simulink model "modelo_rhex_tripode_alterno"  (R2020a)
settings: Solver=VariableStepAuto  StartTime=0.0  StopTime=10.0  RelTol=1e-3
values from neighbouring files (symbols this model uses):
  dist1 = 275    [Parametros_RHex.m]
  espesor = 10    [Parametros_RHex.m]
  masa_C_Leg = 0.057    [Parametros_RHex.m]
  radio = 100    [Parametros_RHex.m]
undefined symbols (not defined in the file or in its folder): X, Y, Z
libraries: sm_lib x34, Contact_Forces_Lib x22, nesl_utility x19, simulink x1
(part 2 of 2)

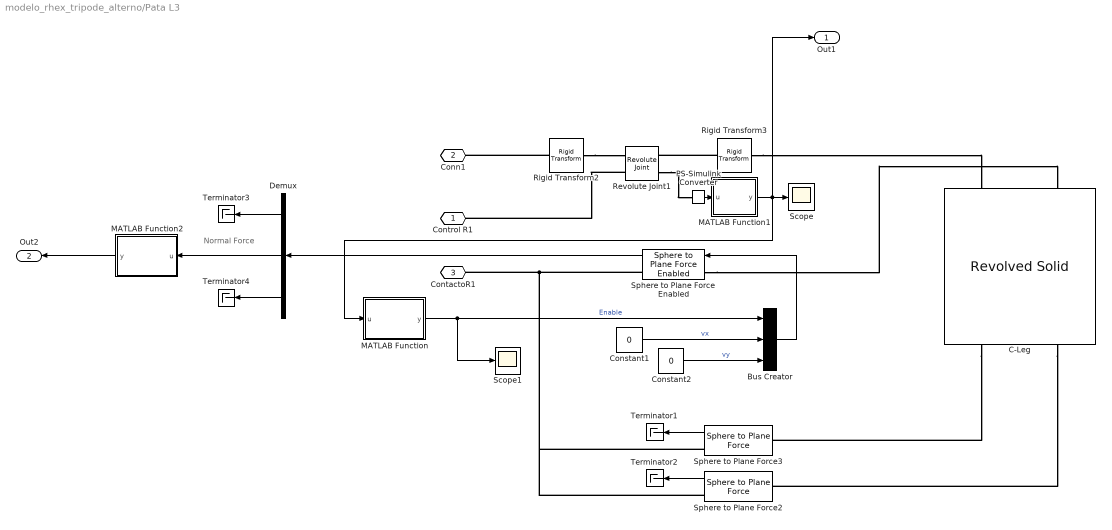
== system modelo_rhex_tripode_alterno/Pata L3 ==
  note: Normal Force
  Bus Creator : BusCreator  Inputs=3
  C-Leg : sm_lib/Body Elements/Revolved Solid  GraphicAmbientColor=[0.15 0.15 0.15 1.0]  BasedOnType=Mass  CenterOfMass=[-42.439/1000 25/1000 -108.743/1000]  CenterOfMassUnits=mm  GraphicDiffuseColor=[1.0 0.2 0.0]  ExportConvexHullGeometry=off  Density=1000  DensityUnits=kg/m^3  DoExposeReferenceFrame=on  GraphicEmissiveColor=[0.0 0.0 0.0 1.0]  ExportEntireGeometry=off  SerializedFrames=<Frames><Frame><Id>Frame1</Id><Value><Name>F1</Name><Origin><Source>GeometricFeature</Source><FeatureName>front point 2</FeatureName></Origin><PrimaryAxis><DefinedDirection>+Z</DefinedDirection><Source>ReferenceFrame</Source><SourceDirection>+Z</SourceDirection><FeatureName></FeatureName></PrimaryAxis><SecondaryAxis><DefinedDirection>+X</DefinedDirection><Source>ReferenceFrame</Source><SourceDirection>+X</SourceDirection><FeatureName></FeatureName></SecondaryAxis></Value></Frame><Frame><Id>Frame2</Id><Value><Name>F2</Name><Origin><Source>GeometricFeature</Source><FeatureName>front point 3</FeatureName></Origin><PrimaryAxis><DefinedDirection>+Z</DefinedDirection><Source>ReferenceFrame</Source><SourceDirection>+Z</SourceDirection><FeatureName></FeatureName></PrimaryAxis><SecondaryAxis><DefinedDirection>+X</DefinedDirection><Source>ReferenceFrame</Source><SourceDirection>+X</SourceDirection><FeatureName></FeatureName></SecondaryAxis></Value></Frame><Frame><Id>Frame3</Id><Value><Name>F3</Name><Origin><Source>GeometricFeature</Source><FeatureName>side surface 2</FeatureName></Origin><PrimaryAxis><DefinedDirection>+Z</DefinedDirection><Source>ReferenceFrame</Source><SourceDirection>+Z</SourceDirection><FeatureName></FeatureName></PrimaryAxis><SecondaryAxis><DefinedDirection>+X</DefinedDirection><Source>ReferenceFrame</Source><SourceDirection>+X</SourceDirection><FeatureName></FeatureName></SecondaryAxis></Value></Frame></Frames>  MarkerShape=Sphere  MarkerSize=10  GraphicType=FromGeometry  InertiaType=Custom  Mass=masa_C_Leg  MassUnits=kg  MomentsOfInertia=[0.001038176 0.000273753 0.001217746]  MomentsOfInertiaUnits=kg*mm^2  GraphicOpacity=1.0  ProductsOfInertia=[-0.000218169 0.000059956 0.000153627]  ProductsOfInertiaUnits=kg*mm^2  RevolutionCrossSection=perfil_C_Leg  RevolutionCrossSectionUnits=mm  RevolutionAngle=240  RevolutionAngleUnits=deg  RevolutionExtent=Custom  GraphicShininess=75  GraphicSpecularColor=[0.5 0.5 0.5 1.0]  GraphicVisPropType=SimpleVisualProperties
  Constant1 : Constant  Value=0
  Constant2 : Constant  Value=0
  Demux : Demux  Outputs=3
  MATLAB Function : MATLAB Function  TreatAsAtomicUnit=on
  MATLAB Function1 : MATLAB Function  TreatAsAtomicUnit=on
  MATLAB Function2 : MATLAB Function  TreatAsAtomicUnit=on
  PS-Simulink Converter : nesl_utility/PS-Simulink Converter  PhysicalDomain=network_engine_domain  SubClassName=ps_output  LeftPortType=input  RightPortType=output  PseudoPeriodic=off  Frequencies=[]  Unit=rad  AffineConversion=off
  Revolute Joint1 : sm_lib/Joints/Revolute Joint  JointMode=Normal  SenseConstraintForce=off  SenseConstraintForceX=off  SenseConstraintForceY=off  SenseConstraintForceZ=off  SenseConstraintTorque=off  SenseConstraintTorqueX=off  SenseConstraintTorqueY=off  SenseConstraintTorqueZ=off  SenseTotalForce=off  SenseTotalForceX=off  SenseTotalForceY=off  SenseTotalForceZ=off  SenseTotalTorque=off  SenseTotalTorqueX=off  SenseTotalTorqueY=off  SenseTotalTorqueZ=off  CompositeWrenchDir=FollowerOnBase  CompositeWrenchFrame=BaseFrame  EquilibriumPosition=0  EquilibriumPositionUnits=deg  SpringStiffness=0  SpringStiffnessUnits=N*m/deg  DampingCoefficient=0  DampingCoefficientUnits=N*m/(deg/s)  TorqueActuationMode=ComputedTorque  MotionActuationMode=InputMotion  SensePosition=on  SenseVelocity=off  SenseAcceleration=off  SenseTorqueForce=off  SenseLowerLimitTorqueForce=off  SenseUpperLimitTorqueForce=off  LowerLimitSpecify=off  LowerLimitBound=-90  LowerLimitBoundUnits=deg  LowerLimitStiffness=1e4  LowerLimitStiffnessUnits=N*m/deg  LowerLimitDamping=10  LowerLimitDampingUnits=N*m/(deg/s)  LowerLimitTransitionRegionWidth=0.1  LowerLimitTransitionRegionWidthUnits=deg  UpperLimitSpecify=off  UpperLimitBound=90  UpperLimitBoundUnits=deg  UpperLimitStiffness=1e4  UpperLimitStiffnessUnits=N*m/deg  UpperLimitDamping=10  UpperLimitDampingUnits=N*m/(deg/s)  UpperLimitTransitionRegionWidth=0.1  UpperLimitTransitionRegionWidthUnits=deg  PositionTargetSpecify=on  PositionTargetPriority=High  PositionTargetValue=180  PositionTargetValueUnits=deg  VelocityTargetSpecify=off  VelocityTargetPriority=High  VelocityTargetValue=0  VelocityTargetValueUnits=deg/s
  Rigid Transform2 : sm_lib/Frames and Transforms/Rigid Transform  TranslationMethod=Cartesian  TranslationStandardOffset=dist4  TranslationLengthUnit=cm  TranslationStandardAxis=+Y  TranslationCartesianOffset=[-23.635 27.496 0]  TranslationROffset=0  TranslationROffsetUnits=m  TranslationZOffset=0  TranslationZOffsetUnits=m  TranslationThetaOffset=0  TranslationThetaOffsetUnits=deg  RotationMethod=StandardAxis  RotationAngleUnits=deg  RotationStandardAxis=+X  RotationAngle=90  RotationArbitraryAxis=[0 0 1]  FollAlignAxisA=-Z  BaseAlignAxisA=+X  FollAlignAxisB=+X  BaseAlignAxisB=+Z  RotationSequenceAxes=FollowerAxes  RotationSequence=XYX  RotationSequenceAngles=[0 0 0]  RotationSequenceAnglesUnits=deg  RotationMatrix=[1 0 0; 0 1 0; 0 0 1]
  Rigid Transform3 : sm_lib/Frames and Transforms/Rigid Transform  TranslationMethod=Cylindrical  TranslationStandardOffset=0  TranslationLengthUnit=mm  TranslationStandardAxis=+Z  TranslationCartesianOffset=[0 -(dist1/2)-radio+(espesor/2) 0]  TranslationROffset=radio-espesor/2  TranslationROffsetUnits=mm  TranslationZOffset=0  TranslationZOffsetUnits=m  TranslationThetaOffset=-120  TranslationThetaOffsetUnits=deg  RotationMethod=StandardAxis  RotationAngleUnits=deg  RotationStandardAxis=+Z  RotationAngle=0  RotationArbitraryAxis=[0 0 1]  FollAlignAxisA=-Z  BaseAlignAxisA=+X  FollAlignAxisB=+X  BaseAlignAxisB=+Z  RotationSequenceAxes=FollowerAxes  RotationSequence=XYX  RotationSequenceAngles=[0 0 0]  RotationSequenceAnglesUnits=deg  RotationMatrix=[1 0 0; 0 1 0; 0 0 1]
  Scope : Scope
  Scope1 : Scope
  Sphere to Plane Force Enabled : Contact_Forces_Lib/3D/Sphere to Plane Force Enabled  sphere_rad=radio/1000  plane_lenx=10  plane_leny=10  plane_depth=0.05/2  force_law=Linear  k_contact=cont1  b_contact=cont2  pen_full_damp_F=0  pen_exponent=1  custom_param_1=1  custom_param_2=1  friction_law=Stick-Slip Continuous  mu_kinetic=fric1  mu_static=fric2  v_thr=0.1  vis_on=off  vis_opc_en=0  vis_len_plaBz=0.005  vis_clr=[0.9 0.2 0.2]  vis_opc=0.7
      settings: SourceProductName=Simscape Multibody Contact Forces Library
  Sphere to Plane Force2 : Contact_Forces_Lib/3D/Sphere to Plane Force  sphere_rad=1e-6  plane_lenx=10  plane_leny=10  plane_depth=0.025  force_law=Linear  k_contact=cont1  b_contact=cont2  pen_full_damp_F=1e-4  pen_exponent=1  custom_param_1=1  custom_param_2=1  friction_law=Stick-Slip Continuous  mu_kinetic=fric1  mu_static=fric2  v_thr=0.1  vis_on=off  vis_opc_en=0  vis_len_plaBz=0.005  vis_clr=[0.9 0.2 0.2]  vis_opc=0.7
  Sphere to Plane Force3 : Contact_Forces_Lib/3D/Sphere to Plane Force  sphere_rad=1e-6  plane_lenx=10  plane_leny=10  plane_depth=0.025  force_law=Linear  k_contact=cont1  b_contact=cont2  pen_full_damp_F=1e-4  pen_exponent=1  custom_param_1=1  custom_param_2=1  friction_law=Stick-Slip Continuous  mu_kinetic=fric1  mu_static=fric2  v_thr=0.1  vis_on=off  vis_opc_en=0  vis_len_plaBz=0.005  vis_clr=[0.9 0.2 0.2]  vis_opc=0.7
  Terminator{1..4} (4 alike) : Terminator
  Control R1 : PMIOPort  Side=Right
  Conn1 : PMIOPort  Port=2  Side=Left
  ContactoR1 : PMIOPort  Port=3  Side=Right
  Out1 : Outport  VectorParamsAs1DForOutWhenUnconnected=off
  Out2 : Outport  Port=2  VectorParamsAs1DForOutWhenUnconnected=off
  wires:
  Constant1/1 -> Bus Creator/2  "vx"
  Constant2/1 -> Bus Creator/3  "vy"
  MATLAB Function/1(y) -> Scope1/1, Bus Creator/1  "Enable"
  PS-Simulink Converter/1 -> MATLAB Function1/1(u)
  MATLAB Function1/1(y) -> Out1/1, MATLAB Function/1(u), Scope/1
  Sphere to Plane Force2/1 -> Terminator2/1
  Sphere to Plane Force3/1 -> Terminator1/1
  Bus Creator/1 -> Sphere to Plane Force Enabled/1
  Demux/1 -> Terminator3/1
  Demux/2 -> MATLAB Function2/1(u)
  Demux/3 -> Terminator4/1
  Sphere to Plane Force Enabled/1 -> Demux/1
  MATLAB Function2/1(y) -> Out2/1
  connections:
  Rigid Transform3/LConn1 -- C-Leg/RConn1
  Rigid Transform3/RConn1 -- Revolute Joint1/RConn1
  Rigid Transform2/LConn1 -- Conn1/RConn1
  Revolute Joint1/LConn2 -- Control R1/RConn1
  Revolute Joint1/RConn2 -- PS-Simulink Converter/LConn1
  C-Leg/LConn1 -- Sphere to Plane Force3/LConn1
  Rigid Transform2/RConn1 -- Revolute Joint1/LConn1
  Sphere to Plane Force2/RConn1 -- Sphere to Plane Force3/RConn1 -- Sphere to Plane Force Enabled/RConn1 -- ContactoR1/RConn1
  C-Leg/LConn2 -- Sphere to Plane Force2/LConn1
  Sphere to Plane Force Enabled/LConn1 -- C-Leg/RConn2

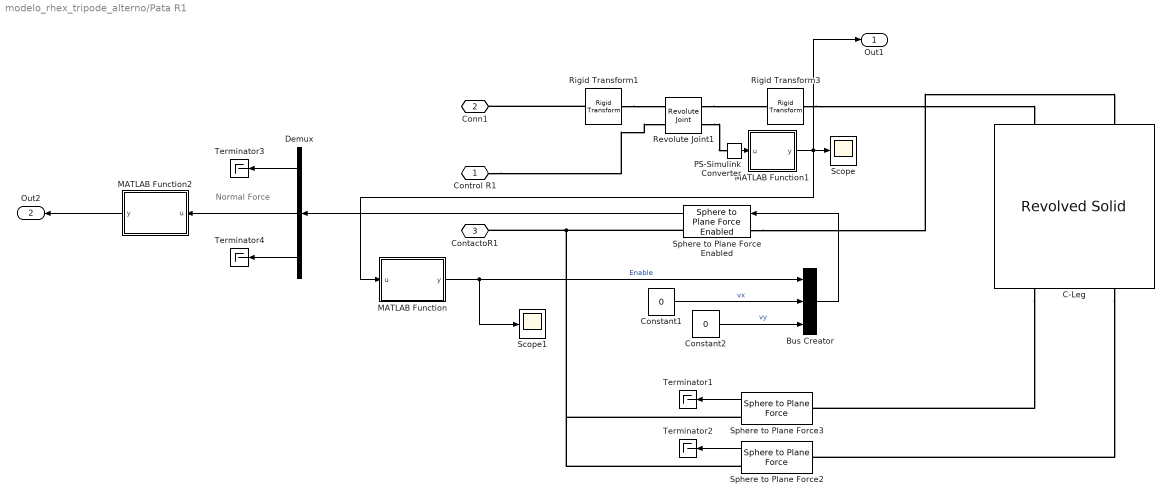
== system modelo_rhex_tripode_alterno/Pata R1 ==
  note: Normal Force
  Bus Creator : BusCreator  Inputs=3
  C-Leg : sm_lib/Body Elements/Revolved Solid  GraphicAmbientColor=[0.15 0.15 0.15 1.0]  BasedOnType=Mass  CenterOfMass=[-42.439/1000 25/1000 -108.743/1000]  CenterOfMassUnits=mm  GraphicDiffuseColor=[1.0 0.2 0.0]  ExportConvexHullGeometry=off  Density=1000  DensityUnits=kg/m^3  DoExposeReferenceFrame=on  GraphicEmissiveColor=[0.0 0.0 0.0 1.0]  ExportEntireGeometry=off  SerializedFrames=<Frames><Frame><Id>Frame1</Id><Value><Name>F1</Name><Origin><Source>GeometricFeature</Source><FeatureName>front point 2</FeatureName></Origin><PrimaryAxis><DefinedDirection>+Z</DefinedDirection><Source>ReferenceFrame</Source><SourceDirection>+Z</SourceDirection><FeatureName></FeatureName></PrimaryAxis><SecondaryAxis><DefinedDirection>+X</DefinedDirection><Source>ReferenceFrame</Source><SourceDirection>+X</SourceDirection><FeatureName></FeatureName></SecondaryAxis></Value></Frame><Frame><Id>Frame2</Id><Value><Name>F2</Name><Origin><Source>GeometricFeature</Source><FeatureName>front point 3</FeatureName></Origin><PrimaryAxis><DefinedDirection>+Z</DefinedDirection><Source>ReferenceFrame</Source><SourceDirection>+Z</SourceDirection><FeatureName></FeatureName></PrimaryAxis><SecondaryAxis><DefinedDirection>+X</DefinedDirection><Source>ReferenceFrame</Source><SourceDirection>+X</SourceDirection><FeatureName></FeatureName></SecondaryAxis></Value></Frame><Frame><Id>Frame3</Id><Value><Name>F3</Name><Origin><Source>GeometricFeature</Source><FeatureName>side surface 2</FeatureName></Origin><PrimaryAxis><DefinedDirection>+Z</DefinedDirection><Source>ReferenceFrame</Source><SourceDirection>+Z</SourceDirection><FeatureName></FeatureName></PrimaryAxis><SecondaryAxis><DefinedDirection>+X</DefinedDirection><Source>ReferenceFrame</Source><SourceDirection>+X</SourceDirection><FeatureName></FeatureName></SecondaryAxis></Value></Frame></Frames>  MarkerShape=Sphere  MarkerSize=10  GraphicType=FromGeometry  InertiaType=Custom  Mass=masa_C_Leg  MassUnits=kg  MomentsOfInertia=[0.001038176 0.000273753 0.001217746]  MomentsOfInertiaUnits=kg*mm^2  GraphicOpacity=1.0  ProductsOfInertia=[-0.000218169 0.000059956 0.000153627]  ProductsOfInertiaUnits=kg*mm^2  RevolutionCrossSection=perfil_C_Leg  RevolutionCrossSectionUnits=mm  RevolutionAngle=240  RevolutionAngleUnits=deg  RevolutionExtent=Custom  GraphicShininess=75  GraphicSpecularColor=[0.5 0.5 0.5 1.0]  GraphicVisPropType=SimpleVisualProperties
  Constant1 : Constant  Value=0
  Constant2 : Constant  Value=0
  Demux : Demux  Outputs=3
  MATLAB Function : MATLAB Function  TreatAsAtomicUnit=on
  MATLAB Function1 : MATLAB Function  TreatAsAtomicUnit=on
  MATLAB Function2 : MATLAB Function  TreatAsAtomicUnit=on
  PS-Simulink Converter : nesl_utility/PS-Simulink Converter  PhysicalDomain=network_engine_domain  SubClassName=ps_output  LeftPortType=input  RightPortType=output  PseudoPeriodic=off  Frequencies=[]  Unit=rad  AffineConversion=off
  Revolute Joint1 : sm_lib/Joints/Revolute Joint  JointMode=Normal  SenseConstraintForce=off  SenseConstraintForceX=off  SenseConstraintForceY=off  SenseConstraintForceZ=off  SenseConstraintTorque=off  SenseConstraintTorqueX=off  SenseConstraintTorqueY=off  SenseConstraintTorqueZ=off  SenseTotalForce=off  SenseTotalForceX=off  SenseTotalForceY=off  SenseTotalForceZ=off  SenseTotalTorque=off  SenseTotalTorqueX=off  SenseTotalTorqueY=off  SenseTotalTorqueZ=off  CompositeWrenchDir=FollowerOnBase  CompositeWrenchFrame=BaseFrame  EquilibriumPosition=0  EquilibriumPositionUnits=deg  SpringStiffness=0  SpringStiffnessUnits=N*m/deg  DampingCoefficient=0  DampingCoefficientUnits=N*m/(deg/s)  TorqueActuationMode=ComputedTorque  MotionActuationMode=InputMotion  SensePosition=on  SenseVelocity=off  SenseAcceleration=off  SenseTorqueForce=off  SenseLowerLimitTorqueForce=off  SenseUpperLimitTorqueForce=off  LowerLimitSpecify=off  LowerLimitBound=-90  LowerLimitBoundUnits=deg  LowerLimitStiffness=1e4  LowerLimitStiffnessUnits=N*m/deg  LowerLimitDamping=10  LowerLimitDampingUnits=N*m/(deg/s)  LowerLimitTransitionRegionWidth=0.1  LowerLimitTransitionRegionWidthUnits=deg  UpperLimitSpecify=off  UpperLimitBound=90  UpperLimitBoundUnits=deg  UpperLimitStiffness=1e4  UpperLimitStiffnessUnits=N*m/deg  UpperLimitDamping=10  UpperLimitDampingUnits=N*m/(deg/s)  UpperLimitTransitionRegionWidth=0.1  UpperLimitTransitionRegionWidthUnits=deg  PositionTargetSpecify=on  PositionTargetPriority=High  PositionTargetValue=180  PositionTargetValueUnits=deg  VelocityTargetSpecify=off  VelocityTargetPriority=High  VelocityTargetValue=0  VelocityTargetValueUnits=deg/s
  Rigid Transform1 : sm_lib/Frames and Transforms/Rigid Transform  TranslationMethod=Cartesian  TranslationStandardOffset=dist4  TranslationLengthUnit=cm  TranslationStandardAxis=+Y  TranslationCartesianOffset=[23.635 -22.425 0]  TranslationROffset=0  TranslationROffsetUnits=m  TranslationZOffset=0  TranslationZOffsetUnits=m  TranslationThetaOffset=0  TranslationThetaOffsetUnits=deg  RotationMethod=StandardAxis  RotationAngleUnits=deg  RotationStandardAxis=+X  RotationAngle=90  RotationArbitraryAxis=[0 0 1]  FollAlignAxisA=-Z  BaseAlignAxisA=+X  FollAlignAxisB=+X  BaseAlignAxisB=+Z  RotationSequenceAxes=FollowerAxes  RotationSequence=XYX  RotationSequenceAngles=[0 0 0]  RotationSequenceAnglesUnits=deg  RotationMatrix=[1 0 0; 0 1 0; 0 0 1]
  Rigid Transform3 : sm_lib/Frames and Transforms/Rigid Transform  TranslationMethod=Cylindrical  TranslationStandardOffset=0  TranslationLengthUnit=mm  TranslationStandardAxis=+Z  TranslationCartesianOffset=[0 -(dist1/2)-radio+(espesor/2) 0]  TranslationROffset=radio-espesor/2  TranslationROffsetUnits=mm  TranslationZOffset=0  TranslationZOffsetUnits=m  TranslationThetaOffset=-120  TranslationThetaOffsetUnits=deg  RotationMethod=StandardAxis  RotationAngleUnits=deg  RotationStandardAxis=+Z  RotationAngle=0  RotationArbitraryAxis=[0 0 1]  FollAlignAxisA=-Z  BaseAlignAxisA=+X  FollAlignAxisB=+X  BaseAlignAxisB=+Z  RotationSequenceAxes=FollowerAxes  RotationSequence=XYX  RotationSequenceAngles=[0 0 0]  RotationSequenceAnglesUnits=deg  RotationMatrix=[1 0 0; 0 1 0; 0 0 1]
  Scope : Scope
  Scope1 : Scope
  Sphere to Plane Force Enabled : Contact_Forces_Lib/3D/Sphere to Plane Force Enabled  sphere_rad=radio/1000  plane_lenx=10  plane_leny=10  plane_depth=0.05/2  force_law=Linear  k_contact=cont1  b_contact=cont2  pen_full_damp_F=0  pen_exponent=1  custom_param_1=1  custom_param_2=1  friction_law=Stick-Slip Continuous  mu_kinetic=fric1  mu_static=fric2  v_thr=0.1  vis_on=off  vis_opc_en=0  vis_len_plaBz=0.005  vis_clr=[0.9 0.2 0.2]  vis_opc=0.7
      settings: SourceProductName=Simscape Multibody Contact Forces Library
  Sphere to Plane Force2 : Contact_Forces_Lib/3D/Sphere to Plane Force  sphere_rad=1e-6  plane_lenx=10  plane_leny=10  plane_depth=0.025  force_law=Linear  k_contact=cont1  b_contact=cont2  pen_full_damp_F=1e-4  pen_exponent=1  custom_param_1=1  custom_param_2=1  friction_law=Stick-Slip Continuous  mu_kinetic=fric1  mu_static=fric2  v_thr=0.1  vis_on=off  vis_opc_en=0  vis_len_plaBz=0.005  vis_clr=[0.9 0.2 0.2]  vis_opc=0.7
  Sphere to Plane Force3 : Contact_Forces_Lib/3D/Sphere to Plane Force  sphere_rad=1e-6  plane_lenx=10  plane_leny=10  plane_depth=0.025  force_law=Linear  k_contact=cont1  b_contact=cont2  pen_full_damp_F=1e-4  pen_exponent=1  custom_param_1=1  custom_param_2=1  friction_law=Stick-Slip Continuous  mu_kinetic=fric1  mu_static=fric2  v_thr=0.1  vis_on=off  vis_opc_en=0  vis_len_plaBz=0.005  vis_clr=[0.9 0.2 0.2]  vis_opc=0.7
  Terminator{1..4} (4 alike) : Terminator
  Control R1 : PMIOPort  Side=Right
  Conn1 : PMIOPort  Port=2  Side=Left
  ContactoR1 : PMIOPort  Port=3  Side=Right
  Out1 : Outport  VectorParamsAs1DForOutWhenUnconnected=off
  Out2 : Outport  Port=2  VectorParamsAs1DForOutWhenUnconnected=off
  wires:
  Constant1/1 -> Bus Creator/2  "vx"
  Constant2/1 -> Bus Creator/3  "vy"
  MATLAB Function/1(y) -> Scope1/1, Bus Creator/1  "Enable"
  PS-Simulink Converter/1 -> MATLAB Function1/1(u)
  MATLAB Function1/1(y) -> Out1/1, MATLAB Function/1(u), Scope/1
  Sphere to Plane Force2/1 -> Terminator2/1
  Sphere to Plane Force3/1 -> Terminator1/1
  Bus Creator/1 -> Sphere to Plane Force Enabled/1
  Demux/1 -> Terminator3/1
  Demux/2 -> MATLAB Function2/1(u)
  Demux/3 -> Terminator4/1
  Sphere to Plane Force Enabled/1 -> Demux/1
  MATLAB Function2/1(y) -> Out2/1
  connections:
  Rigid Transform3/LConn1 -- C-Leg/RConn1
  Rigid Transform1/LConn1 -- Conn1/RConn1
  Control R1/RConn1 -- Revolute Joint1/LConn2
  Sphere to Plane Force2/RConn1 -- Sphere to Plane Force3/RConn1 -- Sphere to Plane Force Enabled/RConn1 -- ContactoR1/RConn1
  C-Leg/LConn1 -- Sphere to Plane Force3/LConn1
  C-Leg/LConn2 -- Sphere to Plane Force2/LConn1
  Revolute Joint1/RConn2 -- PS-Simulink Converter/LConn1
  Revolute Joint1/RConn1 -- Rigid Transform3/RConn1
  Rigid Transform1/RConn1 -- Revolute Joint1/LConn1
  Sphere to Plane Force Enabled/LConn1 -- C-Leg/RConn2

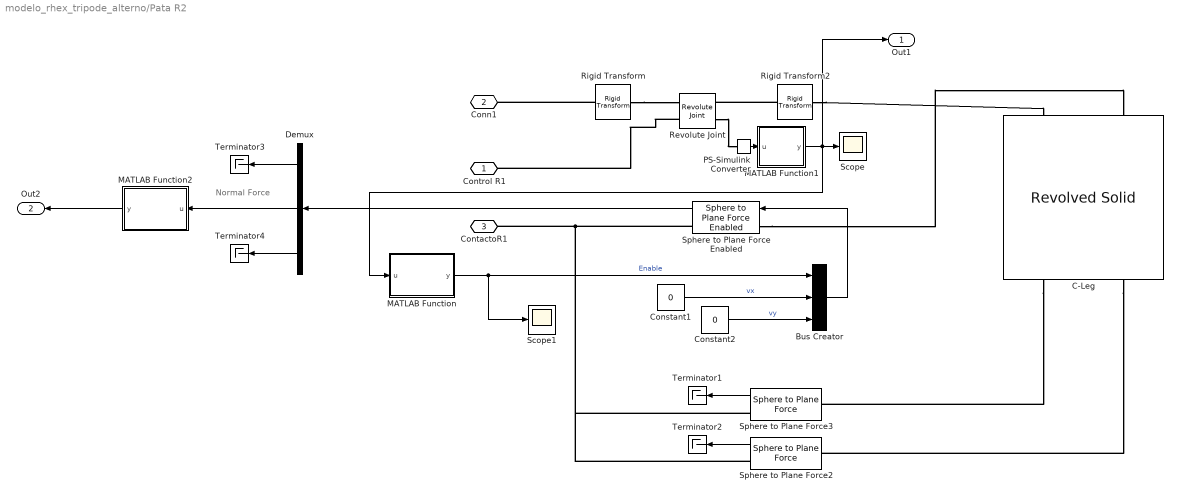
== system modelo_rhex_tripode_alterno/Pata R2 ==
  note: Normal Force
  Bus Creator : BusCreator  Inputs=3
  C-Leg : sm_lib/Body Elements/Revolved Solid  GraphicAmbientColor=[0.15 0.15 0.15 1.0]  BasedOnType=Mass  CenterOfMass=[-42.439/1000 25/1000 -108.743/1000]  CenterOfMassUnits=mm  GraphicDiffuseColor=[1.0 0.2 0.0]  ExportConvexHullGeometry=off  Density=1000  DensityUnits=kg/m^3  DoExposeReferenceFrame=on  GraphicEmissiveColor=[0.0 0.0 0.0 1.0]  ExportEntireGeometry=off  SerializedFrames=<Frames><Frame><Id>Frame1</Id><Value><Name>F1</Name><Origin><Source>GeometricFeature</Source><FeatureName>front point 2</FeatureName></Origin><PrimaryAxis><DefinedDirection>+Z</DefinedDirection><Source>ReferenceFrame</Source><SourceDirection>+Z</SourceDirection><FeatureName></FeatureName></PrimaryAxis><SecondaryAxis><DefinedDirection>+X</DefinedDirection><Source>ReferenceFrame</Source><SourceDirection>+X</SourceDirection><FeatureName></FeatureName></SecondaryAxis></Value></Frame><Frame><Id>Frame2</Id><Value><Name>F2</Name><Origin><Source>GeometricFeature</Source><FeatureName>front point 3</FeatureName></Origin><PrimaryAxis><DefinedDirection>+Z</DefinedDirection><Source>ReferenceFrame</Source><SourceDirection>+Z</SourceDirection><FeatureName></FeatureName></PrimaryAxis><SecondaryAxis><DefinedDirection>+X</DefinedDirection><Source>ReferenceFrame</Source><SourceDirection>+X</SourceDirection><FeatureName></FeatureName></SecondaryAxis></Value></Frame><Frame><Id>Frame3</Id><Value><Name>F3</Name><Origin><Source>GeometricFeature</Source><FeatureName>side surface 2</FeatureName></Origin><PrimaryAxis><DefinedDirection>+Z</DefinedDirection><Source>ReferenceFrame</Source><SourceDirection>+Z</SourceDirection><FeatureName></FeatureName></PrimaryAxis><SecondaryAxis><DefinedDirection>+X</DefinedDirection><Source>ReferenceFrame</Source><SourceDirection>+X</SourceDirection><FeatureName></FeatureName></SecondaryAxis></Value></Frame></Frames>  MarkerShape=Sphere  MarkerSize=10  GraphicType=FromGeometry  InertiaType=Custom  Mass=masa_C_Leg  MassUnits=kg  MomentsOfInertia=[0.001038176 0.000273753 0.001217746]  MomentsOfInertiaUnits=kg*mm^2  GraphicOpacity=1.0  ProductsOfInertia=[-0.000218169 0.000059956 0.000153627]  ProductsOfInertiaUnits=kg*mm^2  RevolutionCrossSection=perfil_C_Leg  RevolutionCrossSectionUnits=mm  RevolutionAngle=240  RevolutionAngleUnits=deg  RevolutionExtent=Custom  GraphicShininess=75  GraphicSpecularColor=[0.5 0.5 0.5 1.0]  GraphicVisPropType=SimpleVisualProperties
  Constant1 : Constant  Value=0
  Constant2 : Constant  Value=0
  Demux : Demux  Outputs=3
  MATLAB Function : MATLAB Function  TreatAsAtomicUnit=on
  MATLAB Function1 : MATLAB Function  TreatAsAtomicUnit=on
  MATLAB Function2 : MATLAB Function  TreatAsAtomicUnit=on
  PS-Simulink Converter : nesl_utility/PS-Simulink Converter  PhysicalDomain=network_engine_domain  SubClassName=ps_output  LeftPortType=input  RightPortType=output  PseudoPeriodic=off  Frequencies=[]  Unit=rad  AffineConversion=off
  Revolute Joint : sm_lib/Joints/Revolute Joint  JointMode=Normal  SenseConstraintForce=off  SenseConstraintForceX=off  SenseConstraintForceY=off  SenseConstraintForceZ=off  SenseConstraintTorque=off  SenseConstraintTorqueX=off  SenseConstraintTorqueY=off  SenseConstraintTorqueZ=off  SenseTotalForce=off  SenseTotalForceX=off  SenseTotalForceY=off  SenseTotalForceZ=off  SenseTotalTorque=off  SenseTotalTorqueX=off  SenseTotalTorqueY=off  SenseTotalTorqueZ=off  CompositeWrenchDir=FollowerOnBase  CompositeWrenchFrame=BaseFrame  EquilibriumPosition=0  EquilibriumPositionUnits=deg  SpringStiffness=0  SpringStiffnessUnits=N*m/deg  DampingCoefficient=0  DampingCoefficientUnits=N*m/(deg/s)  TorqueActuationMode=ComputedTorque  MotionActuationMode=InputMotion  SensePosition=on  SenseVelocity=off  SenseAcceleration=off  SenseTorqueForce=off  SenseLowerLimitTorqueForce=off  SenseUpperLimitTorqueForce=off  LowerLimitSpecify=off  LowerLimitBound=-90  LowerLimitBoundUnits=deg  LowerLimitStiffness=1e4  LowerLimitStiffnessUnits=N*m/deg  LowerLimitDamping=10  LowerLimitDampingUnits=N*m/(deg/s)  LowerLimitTransitionRegionWidth=0.1  LowerLimitTransitionRegionWidthUnits=deg  UpperLimitSpecify=off  UpperLimitBound=90  UpperLimitBoundUnits=deg  UpperLimitStiffness=1e4  UpperLimitStiffnessUnits=N*m/deg  UpperLimitDamping=10  UpperLimitDampingUnits=N*m/(deg/s)  UpperLimitTransitionRegionWidth=0.1  UpperLimitTransitionRegionWidthUnits=deg  PositionTargetSpecify=on  PositionTargetPriority=High  PositionTargetValue=180  PositionTargetValueUnits=deg  VelocityTargetSpecify=off  VelocityTargetPriority=High  VelocityTargetValue=0  VelocityTargetValueUnits=deg/s
  Rigid Transform : sm_lib/Frames and Transforms/Rigid Transform  TranslationMethod=Cartesian  TranslationStandardOffset=dist4  TranslationLengthUnit=cm  TranslationStandardAxis=+Y  TranslationCartesianOffset="[0 -27.135  0]"  TranslationROffset=0  TranslationROffsetUnits=m  TranslationZOffset=0  TranslationZOffsetUnits=m  TranslationThetaOffset=0  TranslationThetaOffsetUnits=deg  RotationMethod=StandardAxis  RotationAngleUnits=deg  RotationStandardAxis=+X  RotationAngle=90  RotationArbitraryAxis=[0 0 1]  FollAlignAxisA=-Z  BaseAlignAxisA=+X  FollAlignAxisB=+X  BaseAlignAxisB=+Z  RotationSequenceAxes=FollowerAxes  RotationSequence=XYX  RotationSequenceAngles=[0 0 0]  RotationSequenceAnglesUnits=deg  RotationMatrix=[1 0 0; 0 1 0; 0 0 1]
  Rigid Transform2 : sm_lib/Frames and Transforms/Rigid Transform  TranslationMethod=Cylindrical  TranslationStandardOffset=0  TranslationLengthUnit=mm  TranslationStandardAxis=+Z  TranslationCartesianOffset=[0 -(dist1/2)-radio+(espesor/2) 0]  TranslationROffset=radio-espesor/2  TranslationROffsetUnits=mm  TranslationZOffset=0  TranslationZOffsetUnits=m  TranslationThetaOffset=-120  TranslationThetaOffsetUnits=deg  RotationMethod=StandardAxis  RotationAngleUnits=deg  RotationStandardAxis=+Z  RotationAngle=0  RotationArbitraryAxis=[0 0 1]  FollAlignAxisA=-Z  BaseAlignAxisA=+X  FollAlignAxisB=+X  BaseAlignAxisB=+Z  RotationSequenceAxes=FollowerAxes  RotationSequence=XYX  RotationSequenceAngles=[0 0 0]  RotationSequenceAnglesUnits=deg  RotationMatrix=[1 0 0; 0 1 0; 0 0 1]
  Scope : Scope
  Scope1 : Scope
  Sphere to Plane Force Enabled : Contact_Forces_Lib/3D/Sphere to Plane Force Enabled  sphere_rad=radio/1000  plane_lenx=10  plane_leny=10  plane_depth=0.05/2  force_law=Linear  k_contact=cont1  b_contact=cont2  pen_full_damp_F=0  pen_exponent=1  custom_param_1=1  custom_param_2=1  friction_law=Stick-Slip Continuous  mu_kinetic=fric1  mu_static=fric2  v_thr=0.1  vis_on=off  vis_opc_en=0  vis_len_plaBz=0.005  vis_clr=[0.9 0.2 0.2]  vis_opc=0.7
      settings: SourceProductName=Simscape Multibody Contact Forces Library
  Sphere to Plane Force2 : Contact_Forces_Lib/3D/Sphere to Plane Force  sphere_rad=1e-6  plane_lenx=10  plane_leny=10  plane_depth=0.025  force_law=Linear  k_contact=cont1  b_contact=cont2  pen_full_damp_F=1e-4  pen_exponent=1  custom_param_1=1  custom_param_2=1  friction_law=Stick-Slip Continuous  mu_kinetic=fric1  mu_static=fric2  v_thr=0.1  vis_on=off  vis_opc_en=0  vis_len_plaBz=0.005  vis_clr=[0.9 0.2 0.2]  vis_opc=0.7
  Sphere to Plane Force3 : Contact_Forces_Lib/3D/Sphere to Plane Force  sphere_rad=1e-6  plane_lenx=10  plane_leny=10  plane_depth=0.025  force_law=Linear  k_contact=cont1  b_contact=cont2  pen_full_damp_F=1e-4  pen_exponent=1  custom_param_1=1  custom_param_2=1  friction_law=Stick-Slip Continuous  mu_kinetic=fric1  mu_static=fric2  v_thr=0.1  vis_on=off  vis_opc_en=0  vis_len_plaBz=0.005  vis_clr=[0.9 0.2 0.2]  vis_opc=0.7
  Terminator{1..4} (4 alike) : Terminator
  Control R1 : PMIOPort  Side=Right
  Conn1 : PMIOPort  Port=2  Side=Left
  ContactoR1 : PMIOPort  Port=3  Side=Right
  Out1 : Outport  VectorParamsAs1DForOutWhenUnconnected=off
  Out2 : Outport  Port=2  VectorParamsAs1DForOutWhenUnconnected=off
  wires:
  Constant1/1 -> Bus Creator/2  "vx"
  Constant2/1 -> Bus Creator/3  "vy"
  MATLAB Function/1(y) -> Scope1/1, Bus Creator/1  "Enable"
  PS-Simulink Converter/1 -> MATLAB Function1/1(u)
  MATLAB Function1/1(y) -> Out1/1, MATLAB Function/1(u), Scope/1
  Sphere to Plane Force2/1 -> Terminator2/1
  Sphere to Plane Force3/1 -> Terminator1/1
  Bus Creator/1 -> Sphere to Plane Force Enabled/1
  Demux/1 -> Terminator3/1
  Demux/2 -> MATLAB Function2/1(u)
  Demux/3 -> Terminator4/1
  Sphere to Plane Force Enabled/1 -> Demux/1
  MATLAB Function2/1(y) -> Out2/1
  connections:
  Rigid Transform2/LConn1 -- C-Leg/RConn1
  Rigid Transform/LConn1 -- Conn1/RConn1
  Revolute Joint/LConn2 -- Control R1/RConn1
  Sphere to Plane Force2/RConn1 -- Sphere to Plane Force3/RConn1 -- Sphere to Plane Force Enabled/RConn1 -- ContactoR1/RConn1
  C-Leg/LConn1 -- Sphere to Plane Force3/LConn1
  C-Leg/LConn2 -- Sphere to Plane Force2/LConn1
  Rigid Transform/RConn1 -- Revolute Joint/LConn1
  Revolute Joint/RConn2 -- PS-Simulink Converter/LConn1
  Rigid Transform2/RConn1 -- Revolute Joint/RConn1
  Sphere to Plane Force Enabled/LConn1 -- C-Leg/RConn2

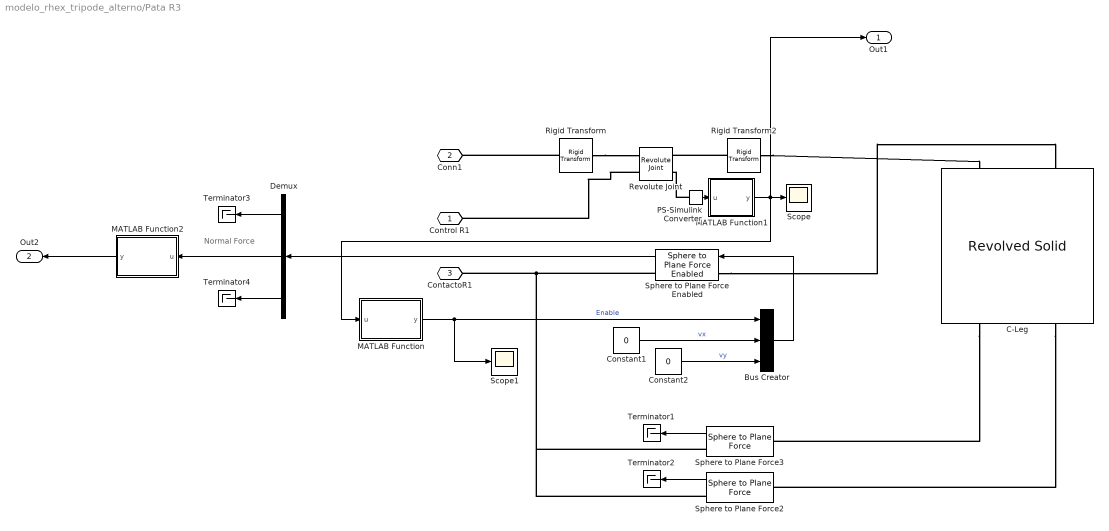
== system modelo_rhex_tripode_alterno/Pata R3 ==
  note: Normal Force
  Bus Creator : BusCreator  Inputs=3
  C-Leg : sm_lib/Body Elements/Revolved Solid  GraphicAmbientColor=[0.15 0.15 0.15 1.0]  BasedOnType=Mass  CenterOfMass=[-42.439/1000 25/1000 -108.743/1000]  CenterOfMassUnits=mm  GraphicDiffuseColor=[1.0 0.2 0.0]  ExportConvexHullGeometry=off  Density=1000  DensityUnits=kg/m^3  DoExposeReferenceFrame=on  GraphicEmissiveColor=[0.0 0.0 0.0 1.0]  ExportEntireGeometry=off  SerializedFrames=<Frames><Frame><Id>Frame1</Id><Value><Name>F1</Name><Origin><Source>GeometricFeature</Source><FeatureName>front point 2</FeatureName></Origin><PrimaryAxis><DefinedDirection>+Z</DefinedDirection><Source>ReferenceFrame</Source><SourceDirection>+Z</SourceDirection><FeatureName></FeatureName></PrimaryAxis><SecondaryAxis><DefinedDirection>+X</DefinedDirection><Source>ReferenceFrame</Source><SourceDirection>+X</SourceDirection><FeatureName></FeatureName></SecondaryAxis></Value></Frame><Frame><Id>Frame2</Id><Value><Name>F2</Name><Origin><Source>GeometricFeature</Source><FeatureName>front point 3</FeatureName></Origin><PrimaryAxis><DefinedDirection>+Z</DefinedDirection><Source>ReferenceFrame</Source><SourceDirection>+Z</SourceDirection><FeatureName></FeatureName></PrimaryAxis><SecondaryAxis><DefinedDirection>+X</DefinedDirection><Source>ReferenceFrame</Source><SourceDirection>+X</SourceDirection><FeatureName></FeatureName></SecondaryAxis></Value></Frame><Frame><Id>Frame3</Id><Value><Name>F3</Name><Origin><Source>GeometricFeature</Source><FeatureName>side surface 2</FeatureName></Origin><PrimaryAxis><DefinedDirection>+Z</DefinedDirection><Source>ReferenceFrame</Source><SourceDirection>+Z</SourceDirection><FeatureName></FeatureName></PrimaryAxis><SecondaryAxis><DefinedDirection>+X</DefinedDirection><Source>ReferenceFrame</Source><SourceDirection>+X</SourceDirection><FeatureName></FeatureName></SecondaryAxis></Value></Frame></Frames>  MarkerShape=Sphere  MarkerSize=10  GraphicType=FromGeometry  InertiaType=Custom  Mass=masa_C_Leg  MassUnits=kg  MomentsOfInertia=[0.001038176 0.000273753 0.001217746]  MomentsOfInertiaUnits=kg*mm^2  GraphicOpacity=1.0  ProductsOfInertia=[-0.000218169 0.000059956 0.000153627]  ProductsOfInertiaUnits=kg*mm^2  RevolutionCrossSection=perfil_C_Leg  RevolutionCrossSectionUnits=mm  RevolutionAngle=240  RevolutionAngleUnits=deg  RevolutionExtent=Custom  GraphicShininess=75  GraphicSpecularColor=[0.5 0.5 0.5 1.0]  GraphicVisPropType=SimpleVisualProperties
  Constant1 : Constant  Value=0
  Constant2 : Constant  Value=0
  Demux : Demux  Outputs=3
  MATLAB Function : MATLAB Function  TreatAsAtomicUnit=on
  MATLAB Function1 : MATLAB Function  TreatAsAtomicUnit=on
  MATLAB Function2 : MATLAB Function  TreatAsAtomicUnit=on
  PS-Simulink Converter : nesl_utility/PS-Simulink Converter  PhysicalDomain=network_engine_domain  SubClassName=ps_output  LeftPortType=input  RightPortType=output  PseudoPeriodic=off  Frequencies=[]  Unit=rad  AffineConversion=off
  Revolute Joint : sm_lib/Joints/Revolute Joint  JointMode=Normal  SenseConstraintForce=off  SenseConstraintForceX=off  SenseConstraintForceY=off  SenseConstraintForceZ=off  SenseConstraintTorque=off  SenseConstraintTorqueX=off  SenseConstraintTorqueY=off  SenseConstraintTorqueZ=off  SenseTotalForce=off  SenseTotalForceX=off  SenseTotalForceY=off  SenseTotalForceZ=off  SenseTotalTorque=off  SenseTotalTorqueX=off  SenseTotalTorqueY=off  SenseTotalTorqueZ=off  CompositeWrenchDir=FollowerOnBase  CompositeWrenchFrame=BaseFrame  EquilibriumPosition=0  EquilibriumPositionUnits=deg  SpringStiffness=0  SpringStiffnessUnits=N*m/deg  DampingCoefficient=0  DampingCoefficientUnits=N*m/(deg/s)  TorqueActuationMode=ComputedTorque  MotionActuationMode=InputMotion  SensePosition=on  SenseVelocity=off  SenseAcceleration=off  SenseTorqueForce=off  SenseLowerLimitTorqueForce=off  SenseUpperLimitTorqueForce=off  LowerLimitSpecify=off  LowerLimitBound=-90  LowerLimitBoundUnits=deg  LowerLimitStiffness=1e4  LowerLimitStiffnessUnits=N*m/deg  LowerLimitDamping=10  LowerLimitDampingUnits=N*m/(deg/s)  LowerLimitTransitionRegionWidth=0.1  LowerLimitTransitionRegionWidthUnits=deg  UpperLimitSpecify=off  UpperLimitBound=90  UpperLimitBoundUnits=deg  UpperLimitStiffness=1e4  UpperLimitStiffnessUnits=N*m/deg  UpperLimitDamping=10  UpperLimitDampingUnits=N*m/(deg/s)  UpperLimitTransitionRegionWidth=0.1  UpperLimitTransitionRegionWidthUnits=deg  PositionTargetSpecify=on  PositionTargetPriority=High  PositionTargetValue=180  PositionTargetValueUnits=deg  VelocityTargetSpecify=off  VelocityTargetPriority=High  VelocityTargetValue=0  VelocityTargetValueUnits=deg/s
  Rigid Transform : sm_lib/Frames and Transforms/Rigid Transform  TranslationMethod=Cartesian  TranslationStandardOffset=dist4  TranslationLengthUnit=cm  TranslationStandardAxis=+Y  TranslationCartesianOffset=[-23.635 -22.425 0]  TranslationROffset=0  TranslationROffsetUnits=m  TranslationZOffset=0  TranslationZOffsetUnits=m  TranslationThetaOffset=0  TranslationThetaOffsetUnits=deg  RotationMethod=StandardAxis  RotationAngleUnits=deg  RotationStandardAxis=+X  RotationAngle=90  RotationArbitraryAxis=[0 0 1]  FollAlignAxisA=-Z  BaseAlignAxisA=+X  FollAlignAxisB=+X  BaseAlignAxisB=+Z  RotationSequenceAxes=FollowerAxes  RotationSequence=XYX  RotationSequenceAngles=[0 0 0]  RotationSequenceAnglesUnits=deg  RotationMatrix=[1 0 0; 0 1 0; 0 0 1]
  Rigid Transform2 : sm_lib/Frames and Transforms/Rigid Transform  TranslationMethod=Cylindrical  TranslationStandardOffset=0  TranslationLengthUnit=mm  TranslationStandardAxis=+Z  TranslationCartesianOffset=[0 -(dist1/2)-radio+(espesor/2) 0]  TranslationROffset=radio-espesor/2  TranslationROffsetUnits=mm  TranslationZOffset=0  TranslationZOffsetUnits=m  TranslationThetaOffset=-120  TranslationThetaOffsetUnits=deg  RotationMethod=StandardAxis  RotationAngleUnits=deg  RotationStandardAxis=+Z  RotationAngle=0  RotationArbitraryAxis=[0 0 1]  FollAlignAxisA=-Z  BaseAlignAxisA=+X  FollAlignAxisB=+X  BaseAlignAxisB=+Z  RotationSequenceAxes=FollowerAxes  RotationSequence=XYX  RotationSequenceAngles=[0 0 0]  RotationSequenceAnglesUnits=deg  RotationMatrix=[1 0 0; 0 1 0; 0 0 1]
  Scope : Scope
  Scope1 : Scope
  Sphere to Plane Force Enabled : Contact_Forces_Lib/3D/Sphere to Plane Force Enabled  sphere_rad=radio/1000  plane_lenx=10  plane_leny=10  plane_depth=0.05/2  force_law=Linear  k_contact=cont1  b_contact=cont2  pen_full_damp_F=0  pen_exponent=1  custom_param_1=1  custom_param_2=1  friction_law=Stick-Slip Continuous  mu_kinetic=fric1  mu_static=fric2  v_thr=0.1  vis_on=off  vis_opc_en=0  vis_len_plaBz=0.005  vis_clr=[0.9 0.2 0.2]  vis_opc=0.7
      settings: SourceProductName=Simscape Multibody Contact Forces Library
  Sphere to Plane Force2 : Contact_Forces_Lib/3D/Sphere to Plane Force  sphere_rad=1e-6  plane_lenx=10  plane_leny=10  plane_depth=0.025  force_law=Linear  k_contact=cont1  b_contact=cont2  pen_full_damp_F=1e-4  pen_exponent=1  custom_param_1=1  custom_param_2=1  friction_law=Stick-Slip Continuous  mu_kinetic=fric1  mu_static=fric2  v_thr=0.1  vis_on=off  vis_opc_en=0  vis_len_plaBz=0.005  vis_clr=[0.9 0.2 0.2]  vis_opc=0.7
  Sphere to Plane Force3 : Contact_Forces_Lib/3D/Sphere to Plane Force  sphere_rad=1e-6  plane_lenx=10  plane_leny=10  plane_depth=0.025  force_law=Linear  k_contact=cont1  b_contact=cont2  pen_full_damp_F=1e-4  pen_exponent=1  custom_param_1=1  custom_param_2=1  friction_law=Stick-Slip Continuous  mu_kinetic=fric1  mu_static=fric2  v_thr=0.1  vis_on=off  vis_opc_en=0  vis_len_plaBz=0.005  vis_clr=[0.9 0.2 0.2]  vis_opc=0.7
  Terminator{1..4} (4 alike) : Terminator
  Control R1 : PMIOPort  Side=Right
  Conn1 : PMIOPort  Port=2  Side=Left
  ContactoR1 : PMIOPort  Port=3  Side=Right
  Out1 : Outport  VectorParamsAs1DForOutWhenUnconnected=off
  Out2 : Outport  Port=2  VectorParamsAs1DForOutWhenUnconnected=off
  wires:
  Constant1/1 -> Bus Creator/2  "vx"
  Constant2/1 -> Bus Creator/3  "vy"
  MATLAB Function/1(y) -> Scope1/1, Bus Creator/1  "Enable"
  PS-Simulink Converter/1 -> MATLAB Function1/1(u)
  MATLAB Function1/1(y) -> Out1/1, MATLAB Function/1(u), Scope/1
  Sphere to Plane Force2/1 -> Terminator2/1
  Sphere to Plane Force3/1 -> Terminator1/1
  Bus Creator/1 -> Sphere to Plane Force Enabled/1
  Demux/1 -> Terminator3/1
  Demux/2 -> MATLAB Function2/1(u)
  Demux/3 -> Terminator4/1
  Sphere to Plane Force Enabled/1 -> Demux/1
  MATLAB Function2/1(y) -> Out2/1
  connections:
  Rigid Transform2/LConn1 -- C-Leg/RConn1
  Rigid Transform/LConn1 -- Conn1/RConn1
  Revolute Joint/LConn2 -- Control R1/RConn1
  Sphere to Plane Force2/RConn1 -- Sphere to Plane Force3/RConn1 -- Sphere to Plane Force Enabled/RConn1 -- ContactoR1/RConn1
  C-Leg/LConn1 -- Sphere to Plane Force3/LConn1
  C-Leg/LConn2 -- Sphere to Plane Force2/LConn1
  PS-Simulink Converter/LConn1 -- Revolute Joint/RConn2
  Rigid Transform2/RConn1 -- Revolute Joint/RConn1
  Rigid Transform/RConn1 -- Revolute Joint/LConn1
  Sphere to Plane Force Enabled/LConn1 -- C-Leg/RConn2

== matlab function modelo_rhex_tripode_alterno/Pata L1/MATLAB Function1 ==
  data: u input; y output
function y = fcn(u)

y = mod(u,2*pi);

== matlab function modelo_rhex_tripode_alterno/Pata L1/MATLAB Function ==
  data: u input; y output
function y = fcn(u)
int8 y
if u>1.43 && u<2.683

    y=0;
else
    y=1;

end

== matlab function modelo_rhex_tripode_alterno/Pata L3/MATLAB Function ==
  data: u input; y output
function y = fcn(u)
int8 y
if u>1.43 && u<2.683

    y=0;
else
    y=1;

end

== matlab function modelo_rhex_tripode_alterno/Pata L3/MATLAB Function1 ==
  data: u input; y output
function y = fcn(u)

y = mod(u,2*pi);

== matlab function modelo_rhex_tripode_alterno/Pata L2/MATLAB Function ==
  data: u input; y output
function y = fcn(u)
int8 y
if u>1.43 && u<2.683

    y=0;
else
    y=1;

end

== matlab function modelo_rhex_tripode_alterno/Pata L2/MATLAB Function1 ==
  data: u input; y output
function y = fcn(u)

y = mod(u,2*pi);

== matlab function modelo_rhex_tripode_alterno/Pata R2/MATLAB Function ==
  data: u input; y output
function y = fcn(u)
int8 y
if u>1.43 && u<2.683

    y=0;
else
    y=1;

end

== matlab function modelo_rhex_tripode_alterno/Pata R2/MATLAB Function1 ==
  data: u input; y output
function y = fcn(u)

y = mod(u,2*pi);

== matlab function modelo_rhex_tripode_alterno/Pata R1/MATLAB Function ==
  data: u input; y output
function y = fcn(u)
int8 y
if u>1.43 && u<2.683

    y=0;
else
    y=1;

end

== matlab function modelo_rhex_tripode_alterno/Pata R1/MATLAB Function1 ==
  data: u input; y output
function y = fcn(u)

y = mod(u,2*pi);

== matlab function modelo_rhex_tripode_alterno/Pata R3/MATLAB Function ==
  data: u input; y output
function y = fcn(u)
int8 y
if u>1.43 && u<2.683

    y=0;
else
    y=1;

end

== matlab function modelo_rhex_tripode_alterno/Pata R3/MATLAB Function1 ==
  data: u input; y output
function y = fcn(u)

y = mod(u,2*pi);

== matlab function modelo_rhex_tripode_alterno/Pata L1/MATLAB Function2 ==
  data: u input; y output
function y = fcn(u)
if u~=0
    y=1;
else
    y=0;

end

== stateflow chart modelo_rhex_tripode_alterno/Chart ==
  state Initial_state
    entry:
    motor_R1_vel = 2;
    motor_R2_vel = 2;
    motor_R3_vel = 2;
    motor_L1_vel = 2;
    motor_L2_vel = 2;
    motor_L3_vel = 2;
  state estado_preparacion
    entry:
    motor_R1_vel = 0;
    motor_R2_vel = 0;
    motor_R3_vel = 0;
    motor_L1_vel = 0;
    motor_L2_vel = 0;
    motor_L3_vel = 0;
  state posicionamiento
    motor_R1_vel = -alpha/2;
    motor_R2_vel = alpha/2;
    motor_R3_vel = -alpha/2;
    motor_L1_vel = alpha/2;
    motor_L2_vel = -alpha/2;
    motor_L3_vel = alpha/2;
  state tripode_2
    motor_R1_vel=(2*pi)-alpha;
    motor_L2_vel=(2*pi)-alpha;
    motor_R3_vel=(2*pi)-alpha;
    motor_L1_vel=alpha;
    motor_R2_vel=alpha;
    motor_L3_vel=alpha;
  state tripode_1
    motor_R1_vel=alpha;
    motor_L2_vel=alpha;
    motor_R3_vel=alpha;
    motor_L1_vel=(2*pi)-alpha;
    motor_R2_vel=(2*pi)-alpha;
    motor_L3_vel=(2*pi)-alpha;
  (default) -> Initial_state
  Initial_state -> estado_preparacion : [(Pos_R1<=3.647)]
  estado_preparacion -> posicionamiento : [(motor_R1_vel==0)]
  posicionamiento -> tripode_1 : [after(1,sec)]
  tripode_2 -> tripode_1 : [after(1,sec)]
  tripode_1 -> tripode_2 : [after(1,sec)]
  data: Pos_R1 input; Pos_R3 input; Pos_R2 input; Pos_L2 input; Pos_L1 input; Pos_L3 input; motor_L1_vel output; motor_L2_vel output; motor_R3_vel output; motor_R1_vel output; motor_R2_vel output; motor_L3_vel output; TR1 input; TR2 input; TR3 input; TL1 input; TL2 input; TL3 input; alpha input

== matlab function modelo_rhex_tripode_alterno/Pata L3/MATLAB Function2 ==
  data: u input; y output
function y = fcn(u)
if u~=0
    y=1;
else
    y=0;

end

== matlab function modelo_rhex_tripode_alterno/Pata L2/MATLAB Function2 ==
  data: u input; y output
function y = fcn(u)
if u~=0
    y=1;
else
    y=0;

end

== matlab function modelo_rhex_tripode_alterno/Pata R2/MATLAB Function2 ==
  data: u input; y output
function y = fcn(u)
if u~=0
    y=1;
else
    y=0;

end

== matlab function modelo_rhex_tripode_alterno/Pata R1/MATLAB Function2 ==
  data: u input; y output
function y = fcn(u)
if u~=0
    y=1;
else
    y=0;

end

== matlab function modelo_rhex_tripode_alterno/Pata R3/MATLAB Function2 ==
  data: u input; y output
function y = fcn(u)
if u~=0
    y=1;
else
    y=0;

end
